simulink library "LIB_TF_G_113"  (Simulink 8.6)
settings: Solver=ode45  StartTime=0.0  StopTime=10.0  RelTol=1e-3
PreLoadFcn:
  | if exist('tl_preloadfcn','file'), tl_preloadfcn(gcs,402); end
PostLoadFcn:
  | if exist('tl_postloadfcn','file'), tl_postloadfcn(gcs,402); end
undefined symbols (not defined in the file or in its folder): ddv
CloseFcn:
  | if exist('tl_closefcn','file'), tl_closefcn(gcs); end
settings Model: TLRevision=402  Creator=cedric.sauvage  LastModifiedBy=pierre-olivier.pilot

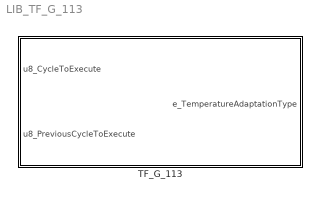
== system LIB_TF_G_113 ==
  TF_G_113 : Subsystem  TreatAsAtomicUnit=on

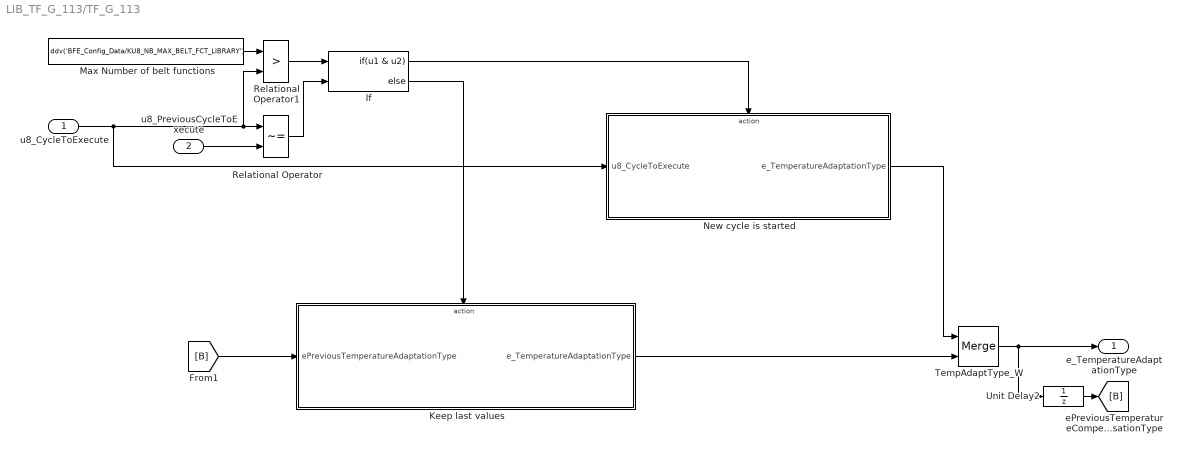
== system LIB_TF_G_113/TF_G_113 ==
  u8_CycleToExecute : Inport
  u8_PreviousCycleToExecute : Inport  Port=2
  If : If  NumInputs=2  IfExpression=u1 & u2
  Keep last values : Subsystem  TreatAsAtomicUnit=on
  Max Number of belt functions : Constant  Value=ddv('BFE_Config_Data/KU8_NB_MAX_BELT_FCT_LIBRARY')  mask(TL_Constant){data={'output',{'variable','BFE_Config_Data/KU8_NB_MAX_BELT_FCT_LIBRARY'},'date',735951.66822505789}}
      settings: CopyFcn=if exist('tl_reset_reviewflag','file')==2,tl_reset_reviewflag(gcbh);end  DeleteFcn=if exist('delete_tlblock','file')==2,delete_tlblock(gcbh);end  NameChangeFcn=if exist('rename_tlblock','file')==2,rename_tlblock(gcbh);end  OpenFcn=if exist('tl_open_blockdlg','file')==2,tl_open_blockdlg(gcbh);else,open_system(gcbh,'parameter');end
      mask Help: eval(['if exist(''tl_online_help'',''file'') == 2, tl_online_help(''Topic'',''TL_Constant''),else, web([''jar:file:///'',matlabroot,''/help/toolbox/simulink/help.jar!/slref/' lower(get_param(gcbh,'Blocktype')) '.html''], ''-helpbrowser''),end'])
      mask Display: plot([-0.05, 1.05, NaN, -0.05, 1.05],[.01, .01, NaN, .99, .99])
  New cycle is started : Subsystem  TreatAsAtomicUnit=on
  Relational Operator : RelationalOperator  Operator=~=  OutDataTypeStr=boolean  mask(TL_RelationalOperator){data={'date',735951.66814618057}}
      settings: DeleteFcn=if exist('delete_tlblock','file')==2,delete_tlblock(gcbh);end  NameChangeFcn=if exist('rename_tlblock','file')==2,rename_tlblock(gcbh);end  OpenFcn=if exist('tl_open_blockdlg','file')==2,tl_open_blockdlg(gcbh);else,open_system(gcbh,'parameter');end
      mask Help: eval(['if exist(''tl_online_help'',''file'') == 2, tl_online_help(''Topic'',''TL_RelationalOperator''),else, web([''jar:file:///'',matlabroot,''/help/toolbox/simulink/help.jar!/slref/' lower(get_param(gcbh,'Blocktype')) '.html''], ''-helpbrowser''),end'])
      mask Display: plot([-0.05, 1.05, NaN, -0.05, 1.05],[.01, .01, NaN, .99, .99])
  Relational Operator1 : RelationalOperator  Operator=>  OutDataTypeStr=boolean  mask(TL_RelationalOperator){data={'date',735951.6681459375}}
      settings: DeleteFcn=if exist('delete_tlblock','file')==2,delete_tlblock(gcbh);end  NameChangeFcn=if exist('rename_tlblock','file')==2,rename_tlblock(gcbh);end  OpenFcn=if exist('tl_open_blockdlg','file')==2,tl_open_blockdlg(gcbh);else,open_system(gcbh,'parameter');end
      mask Help: eval(['if exist(''tl_online_help'',''file'') == 2, tl_online_help(''Topic'',''TL_RelationalOperator''),else, web([''jar:file:///'',matlabroot,''/help/toolbox/simulink/help.jar!/slref/' lower(get_param(gcbh,'Blocktype')) '.html''], ''-helpbrowser''),end'])
      mask Display: plot([-0.05, 1.05, NaN, -0.05, 1.05],[.01, .01, NaN, .99, .99])
  TempAdaptType_W : Merge  InitialOutput=0  mask(TL_Merge){data={'logdata',{'loggingmode',1},'output',{'name','eTemperatureCompensationType','type','UInt8','inheritscaling',0},'date',735951.6681456482}}
      settings: CopyFcn=if exist('tl_reset_reviewflag','file')==2,tl_reset_reviewflag(gcbh);end  DeleteFcn=if exist('delete_tlblock','file')==2,delete_tlblock(gcbh);end  NameChangeFcn=if exist('rename_tlblock','file')==2,rename_tlblock(gcbh);end  OpenFcn=if exist('tl_open_blockdlg','file')==2,tl_open_blockdlg(gcbh);else,open_system(gcbh,'parameter');end
      mask Help: eval(['if exist(''tl_online_help'',''file'') == 2, tl_online_help(''Topic'',''TL_Merge''),else, web([''jar:file:///'',matlabroot,''/help/toolbox/simulink/help.jar!/slref/' lower(get_param(gcbh,'Blocktype')) '.html''], ''-helpbrowser''),end'])
      mask Display: plot([-0.05, 1.05, NaN, -0.05, 1.05],[.01, .01, NaN, .99, .99])
  Unit Delay2 : UnitDelay  SampleTime=-1  mask(TL_UnitDelay){data={'output',{'type','UInt8'},'state',{'name','ePreviousCompensationType','type','UInt8'},'date',735951.66814369208}}
      settings: CopyFcn=if exist('tl_reset_reviewflag','file')==2,tl_reset_reviewflag(gcbh);end  DeleteFcn=if exist('delete_tlblock','file')==2,delete_tlblock(gcbh);end  NameChangeFcn=if exist('rename_tlblock','file')==2,rename_tlblock(gcbh);end  OpenFcn=if exist('tl_open_blockdlg','file')==2,tl_open_blockdlg(gcbh);else,open_system(gcbh,'parameter');end
      mask Help: eval(['if exist(''tl_online_help'',''file'') == 2, tl_online_help(''Topic'',''TL_UnitDelay''),else, web([''jar:file:///'',matlabroot,''/help/toolbox/simulink/help.jar!/slref/' lower(get_param(gcbh,'Blocktype')) '.html''], ''-helpbrowser''),end'])
      mask Display: plot([-0.05, 1.05, NaN, -0.05, 1.05],[.01, .01, NaN, .99, .99])
  e_TemperatureAdaptationType : Outport
  wires:
  u8_CycleToExecute/1 -> Relational Operator/1, Relational Operator1/2, New cycle is started/1(u8_CycleToExecute)
  Max Number of belt functions/1 -> Relational Operator1/1
  If/1 -> New cycle is started/Action
  Relational Operator1/1 -> If/1
  Relational Operator/1 -> If/2
  If/2 -> Keep last values/Action
  Keep last values/1(e_TemperatureAdaptationType) -> TempAdaptType_W/2
  New cycle is started/1(e_TemperatureAdaptationType) -> TempAdaptType_W/1
  TempAdaptType_W/1 -> e_TemperatureAdaptationType/1, Unit Delay2/1
  Unit Delay2/1 -> [B]
  [B] -> Keep last values/1(ePreviousTemperatureAdaptationType)
  u8_PreviousCycleToExecute/1 -> Relational Operator/2

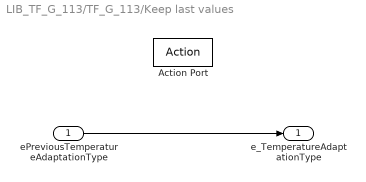
== system LIB_TF_G_113/TF_G_113/Keep last values ==
  ePreviousTemperatureAdaptationType : Inport
  Action Port : ActionPort  ActionType=else
  e_TemperatureAdaptationType : Outport  InitialOutput=0
  wires:
  ePreviousTemperatureAdaptationType/1 -> e_TemperatureAdaptationType/1

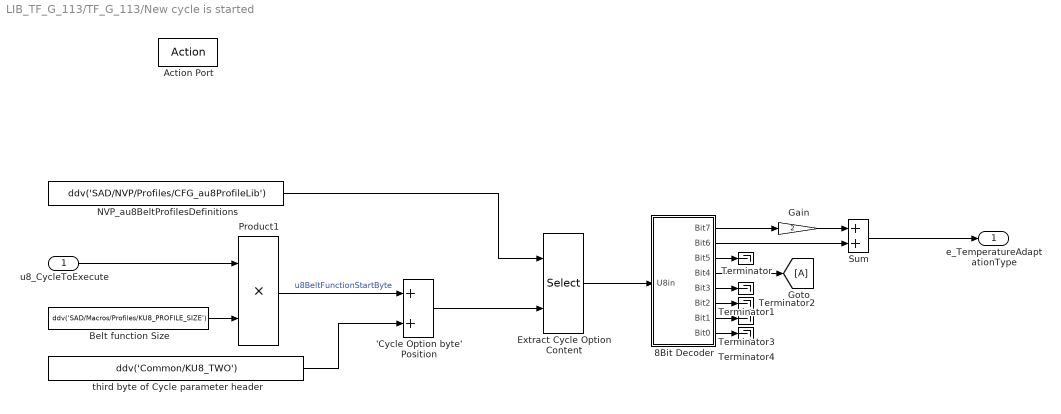
== system LIB_TF_G_113/TF_G_113/New cycle is started ==
  u8_CycleToExecute : Inport
  Action Port : ActionPort
  'Cycle Option byte' Position : Sum  RequirementInfo={} %GIDa_7880887a_88ef_4820_ba37_f9cacbb46ca1  SaturateOnIntegerOverflow=on  OutDataTypeStr=Inherit: Same as first input  mask(TL_Sum){data={'output',{'name','u8CycleOptionBytePos','type','UInt8'},'date',735951.66822467593}}
      settings: CopyFcn=if exist('tl_reset_reviewflag','file')==2,tl_reset_reviewflag(gcbh);end  DeleteFcn=if exist('delete_tlblock','file')==2,delete_tlblock(gcbh);end  NameChangeFcn=if exist('rename_tlblock','file')==2,rename_tlblock(gcbh);end  OpenFcn=if exist('tl_open_blockdlg','file')==2,tl_open_blockdlg(gcbh);else,open_system(gcbh,'parameter');end
      mask Help: eval(['if exist(''tl_online_help'',''file'') == 2, tl_online_help(''Topic'',''TL_Sum''),else, web([''jar:file:///'',matlabroot,''/help/toolbox/simulink/help.jar!/slref/' lower(get_param(gcbh,'Blocktype')) '.html''], ''-helpbrowser''),end'])
      mask Display: plot([-0.05, 1.05, NaN, -0.05, 1.05],[.01, .01, NaN, .99, .99])
  8Bit Decoder : Subsystem  mask(TLSAMPLES_8BIT_DECODER){}
      mask help:
      | Decodes one UInt8 byte into 8 bits.
      | All inputs are boolean variables.
      |
      | Sample implementation using TargetLink Custom Code block.
      | Version 1.0.
  Belt function Size : Constant  RequirementInfo={} %GIDa_4d2af6e9_43d8_48cb_a10a_6f19e343c165  Value=ddv('SAD/Macros/Profiles/KU8_PROFILE_SIZE')  OutDataTypeStr=Inherit: Inherit via back propagation  mask(TL_Constant){data={'output',{'variable','SAD/Macros/Profiles/KU8_PROFILE_SIZE'},'date',738321.57783990738}}
      settings: CopyFcn=if exist('tl_reset_reviewflag','file')==2,tl_reset_reviewflag(gcbh);end  DeleteFcn=if exist('delete_tlblock','file')==2,delete_tlblock(gcbh);end  NameChangeFcn=if exist('rename_tlblock','file')==2,rename_tlblock(gcbh);end  OpenFcn=if exist('tl_open_blockdlg','file')==2,tl_open_blockdlg(gcbh);else,open_system(gcbh,'parameter');end
      mask Help: eval(['if exist(''tl_online_help'',''file'') == 2, tl_online_help(''Topic'',''TL_Constant''),else, web([''jar:file:///'',matlabroot,''/help/toolbox/simulink/help.jar!/slref/' lower(get_param(gcbh,'Blocktype')) '.html''], ''-helpbrowser''),end'])
      mask Display: plot([-0.05, 1.05, NaN, -0.05, 1.05],[.01, .01, NaN, .99, .99])
  Extract Cycle Option Content : Selector  RequirementInfo={} %GIDa_c4b93e9e_9e61_442f_aace_a8e944c66281  IndexMode=Zero-based  IndexOptions=Index vector (port)  Indices=[1:3]  OutputSizes=1
  Gain : Gain  Gain=2  mask(TL_Gain){data={'output',{'type','UInt8'},'date',735951.66815128468}}
      settings: CopyFcn=if exist('tl_reset_reviewflag','file')==2,tl_reset_reviewflag(gcbh);end  DeleteFcn=if exist('delete_tlblock','file')==2,delete_tlblock(gcbh);end  NameChangeFcn=if exist('rename_tlblock','file')==2,rename_tlblock(gcbh);end  OpenFcn=if exist('tl_open_blockdlg','file')==2,tl_open_blockdlg(gcbh);else,open_system(gcbh,'parameter');end
      mask Help: eval(['if exist(''tl_online_help'',''file'') == 2, tl_online_help(''Topic'',''TL_Gain''),else, web([''jar:file:///'',matlabroot,''/help/toolbox/simulink/help.jar!/slref/' lower(get_param(gcbh,'Blocktype')) '.html''], ''-helpbrowser''),end'])
      mask Display: plot([0, .9, 0],[.05, .5, .95])
  NVP_au8BeltProfilesDefinitions : Constant  RequirementInfo={} %GIDa_64a44852_3452_4006_91db_d2eae2d4123a  Value=ddv('SAD/NVP/Profiles/CFG_au8ProfileLib')  OutDataTypeStr=uint8  SampleTime=-1  mask(TL_Constant){data={'output',{'variable','SAD/NVP/Profiles/CFG_au8ProfileLib'},'autoscaling',{'mode',2,'scalingvalid',1},'date',738321.57767927088}}
      settings: CopyFcn=if exist('tl_reset_reviewflag','file')==2,tl_reset_reviewflag(gcbh);end  DeleteFcn=if exist('delete_tlblock','file')==2,delete_tlblock(gcbh);end  NameChangeFcn=if exist('rename_tlblock','file')==2,rename_tlblock(gcbh);end  OpenFcn=if exist('tl_open_blockdlg','file')==2,tl_open_blockdlg(gcbh);else,open_system(gcbh,'parameter');end
      mask Help: eval(['if exist(''tl_online_help'',''file'') == 2, tl_online_help(''Topic'',''TL_Constant''),else, web([''jar:file:///'',matlabroot,''/help/toolbox/simulink/help.jar!/slref/' lower(get_param(gcbh,'Blocktype')) '.html''], ''-helpbrowser''),end'])
      mask Display: plot([-0.05, 1.05, NaN, -0.05, 1.05],[.01, .01, NaN, .99, .99])
  Product1 : Product  RequirementInfo={} %GIDa_10c25ed2_85fd_4f5d_af58_9e981fb8d77e  OutDataTypeStr=uint8  SaturateOnIntegerOverflow=on  RndMeth=Zero  mask(TL_Product){data={'output',{'type','UInt8'},'date',735951.66814782412}}
      settings: CopyFcn=if exist('tl_reset_reviewflag','file')==2,tl_reset_reviewflag(gcbh);end  DeleteFcn=if exist('delete_tlblock','file')==2,delete_tlblock(gcbh);end  NameChangeFcn=if exist('rename_tlblock','file')==2,rename_tlblock(gcbh);end  OpenFcn=if exist('tl_open_blockdlg','file')==2,tl_open_blockdlg(gcbh);else,open_system(gcbh,'parameter');end
      mask Help: eval(['if exist(''tl_online_help'',''file'') == 2, tl_online_help(''Topic'',''TL_Product''),else, web([''jar:file:///'',matlabroot,''/help/toolbox/simulink/help.jar!/slref/' lower(get_param(gcbh,'Blocktype')) '.html''], ''-helpbrowser''),end'])
      mask Display: plot([-0.05, 1.05, NaN, -0.05, 1.05],[.01, .01, NaN, .99, .99])
  Sum : Sum  mask(TL_Sum){data={'output',{'type','UInt8'},'date',735951.66814744216}}
      settings: CopyFcn=if exist('tl_reset_reviewflag','file')==2,tl_reset_reviewflag(gcbh);end  DeleteFcn=if exist('delete_tlblock','file')==2,delete_tlblock(gcbh);end  NameChangeFcn=if exist('rename_tlblock','file')==2,rename_tlblock(gcbh);end  OpenFcn=if exist('tl_open_blockdlg','file')==2,tl_open_blockdlg(gcbh);else,open_system(gcbh,'parameter');end
      mask Help: eval(['if exist(''tl_online_help'',''file'') == 2, tl_online_help(''Topic'',''TL_Sum''),else, web([''jar:file:///'',matlabroot,''/help/toolbox/simulink/help.jar!/slref/' lower(get_param(gcbh,'Blocktype')) '.html''], ''-helpbrowser''),end'])
      mask Display: plot([-0.05, 1.05, NaN, -0.05, 1.05],[.01, .01, NaN, .99, .99])
  Terminator{,1..4} (5 alike) : Terminator
  third byte of Cycle parameter header : Constant  RequirementInfo={} %GIDa_6d8be3d5_af2b_4d00_8d5e_2adc9650b4bc  Value=ddv('Common/KU8_TWO')  OutDataTypeStr=uint8  mask(TL_Constant){data={'output',{'variable','Common/KU8_TWO'},'date',735951.66814704856}}
      settings: CopyFcn=if exist('tl_reset_reviewflag','file')==2,tl_reset_reviewflag(gcbh);end  DeleteFcn=if exist('delete_tlblock','file')==2,delete_tlblock(gcbh);end  NameChangeFcn=if exist('rename_tlblock','file')==2,rename_tlblock(gcbh);end  OpenFcn=if exist('tl_open_blockdlg','file')==2,tl_open_blockdlg(gcbh);else,open_system(gcbh,'parameter');end
      mask Help: eval(['if exist(''tl_online_help'',''file'') == 2, tl_online_help(''Topic'',''TL_Constant''),else, web([''jar:file:///'',matlabroot,''/help/toolbox/simulink/help.jar!/slref/' lower(get_param(gcbh,'Blocktype')) '.html''], ''-helpbrowser''),end'])
      mask Display: plot([-0.05, 1.05, NaN, -0.05, 1.05],[.01, .01, NaN, .99, .99])
  e_TemperatureAdaptationType : Outport  InitialOutput=0
  wires:
  Product1/1 -> 'Cycle Option byte' Position/1  "u8BeltFunctionStartByte"
  Belt function Size/1 -> Product1/2
  third byte of Cycle parameter header/1 -> 'Cycle Option byte' Position/2
  u8_CycleToExecute/1 -> Product1/1
  NVP_au8BeltProfilesDefinitions/1 -> Extract Cycle Option Content/1
  'Cycle Option byte' Position/1 -> Extract Cycle Option Content/2
  Extract Cycle Option Content/1 -> 8Bit Decoder/1(U8in)
  8Bit Decoder/3(Bit5) -> Terminator/1
  8Bit Decoder/8(Bit0) -> Terminator4/1
  8Bit Decoder/7(Bit1) -> Terminator3/1
  8Bit Decoder/6(Bit2) -> Terminator2/1
  8Bit Decoder/5(Bit3) -> Terminator1/1
  8Bit Decoder/1(Bit7) -> Gain/1
  Gain/1 -> Sum/1
  8Bit Decoder/2(Bit6) -> Sum/2
  Sum/1 -> e_TemperatureAdaptationType/1
  8Bit Decoder/4(Bit4) -> [A]

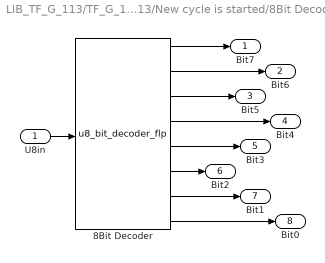
== system LIB_TF_G_113/TF_G_113/New cycle is started/8Bit Decoder ==
  U8in : Inport
  8Bit Decoder : S-Function  FunctionName=u8_bit_decoder_flp  Parameters=dt  SFunctionDeploymentMode=off  EnableBusSupport=off  mask(TL_CustomCode){data={'#state',0,'#param',0,'#work',0,'#output',8,'#logdata',8,'codefile','u8_bit_decoder.c','output#1',{'name','u8TemperatureAdaptB7','varname','bit7','type','Bool'},'output#2',{'name','u8TemperatureAdaptB6','varname','bit6','type','Bool'},'output#3',{'name','bUnused_bit5','varname','bit5','type','Bool'},'output#4',{'name','bIsPowerDegradableCycle','varname','bit4','type','Bool'},'output#5',{'name','bUnused_bit3','varname','bit3','type','Bool'},'output#6',{'name','bUnused_bit2','varname','bit2','type','Bool'},'output#7',{'name','bUnused_bit1','varname','bit1','type','Bool'},'output#8',{'name','bUnused_bit0','varname','bit0','type','Bool'},'input',{'name','$S_$B_in','varname','u8in','type','UInt8'},'date',735951.66822387732}, dt=-1}
      mask help:
      | TargetLink Custom Code block:
      | Allows to insert custom code into a TargetLink application.
      settings: DeleteFcn=if exist('delete_tlblock','file')==2,delete_tlblock(gcbh);end  NameChangeFcn=if exist('rename_tlblock','file')==2,rename_tlblock(gcbh);end  OpenFcn=if exist('tl_open_blockdlg','file')==2,tl_open_blockdlg(gcbh);else,open_system(gcbh,'mask');end
      mask Help: eval('if exist(''tl_online_help'',''file'') == 2, tl_online_help(''Topic'',get_param(gcbh,''MaskType'')),end')
      mask Display:
      | plot([-0.05, 1.05, NaN, -0.05, 1.05],[.01, .01, NaN, .99, .99])
      | ; disp('u8_bit_decoder.c');port_label('input',1,'u8in');port_label('output',1,'bit7');port_label('output',2,'bit6');port_label('output',3,'bit5');port_label('output',4,'bit4');port_label('output',5,'bit3');port_label('output',6,'bit2');port_label('output',7,'bit1');port_label('output',8,'bit0');
  Bit7 : Outport
  Bit6 : Outport  Port=2
  Bit5 : Outport  Port=3
  Bit4 : Outport  Port=4
  Bit3 : Outport  Port=5
  Bit2 : Outport  Port=6
  Bit1 : Outport  Port=7
  Bit0 : Outport  Port=8
  wires:
  8Bit Decoder/8 -> Bit0/1
  8Bit Decoder/7 -> Bit1/1
  8Bit Decoder/5 -> Bit3/1
  8Bit Decoder/4 -> Bit4/1
  8Bit Decoder/3 -> Bit5/1
  8Bit Decoder/2 -> Bit6/1
  8Bit Decoder/1 -> Bit7/1
  8Bit Decoder/6 -> Bit2/1
  U8in/1 -> 8Bit Decoder/1
